simulink model "Problem2"  (R2017a)
settings: Solver=ode45  StartTime=0.0  StopTime=10.0  MaxStep=0.001  MinStep=0.0001  RelTol=1e-5
settings Model: Creator=Gowtham  LastModifiedBy=Gowtham

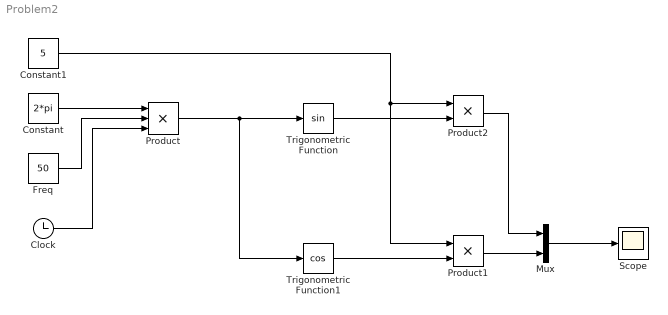
== system Problem2 ==
  Clock : Clock
  Constant : Constant  Value=2*pi
  Constant1 : Constant  Value=5
  Freq : Constant  Value=50
  Mux : Mux  Inputs=2
  Product : Product  Inputs=3
  Product1 : Product
  Product2 : Product
  Scope : Scope
  Trigonometric Function : Trigonometry
  Trigonometric Function1 : Trigonometry  Operator=cos
  wires:
  Freq/1 -> Product/2
  Constant/1 -> Product/1
  Clock/1 -> Product/3
  Product/1 -> Trigonometric Function1/1, Trigonometric Function/1
  Trigonometric Function1/1 -> Product1/2
  Constant1/1 -> Product1/1, Product2/1
  Product2/1 -> Mux/1
  Product1/1 -> Mux/2
  Mux/1 -> Scope/1
  Trigonometric Function/1 -> Product2/2
